simulink model "TunedFuzzy"  (R2024a)
settings: Solver=VariableStepAuto  StartTime=0.0  StopTime=0.24  RelTol=1e-3
InitFcn:
  | fsw = 1e6;
  | Tsw = 1/fsw;
  | 
  | fs = 10e3;%fsw / 4;
  | Ts = 1/fs;
StopFcn:
  | MAE = mean(abs(out.E));
  | Eta = sum((out.P_Pmax{1}.Values.Data))/sum(out.P_Pmax{2}.Values.Data);
undefined symbols (not defined in the file or in its folder): Ion, Lithium, result_Extrapolated_copy
libraries: spsSeriesRLCBranchLib x5, spsCurrentMeasurementLib x4, spsMosfetLib x4, spsVoltageMeasurementLib x3, spsDiodeLib x2, spsBatteryLib x1, spsControlledCurrentSourceLib x1, fuzblock x1, spsPWMGeneratorDCDCLib x1, SignalEditorBlockLib x1, sps_lib x1
settings Model: Creator=kimiaahmadi  LastModifiedBy=kimiaahmadi

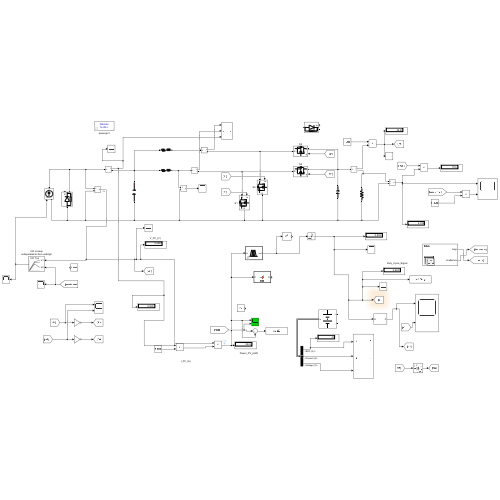
[thumbnail: Simulink's stored preview of the top-level diagram]
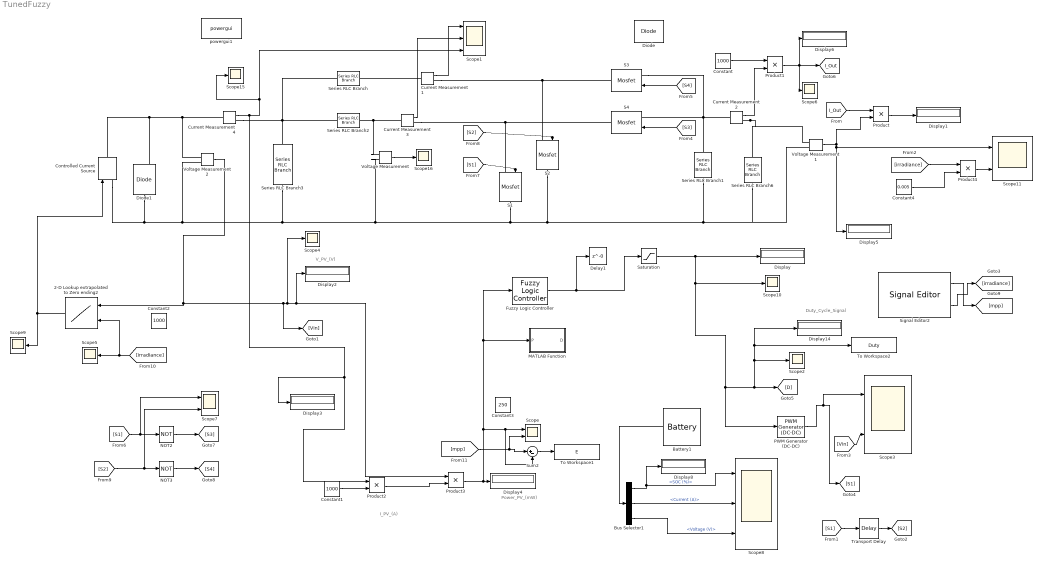
== system TunedFuzzy ==
  note: V_PV_(V)
  note: Duty_Cycle_Signal
  note: I_PV_(A)
  note: Power_PV_(mW)
  2-D Lookup extrapolated to Zero ending2 : Lookup_n-D  BreakpointsForDimension1=[0:7.058900000000000e-04:0.611]  BreakpointsForDimension2=[1:1000]  Table=[result_Extrapolated_copy].'  ExtrapMethod=Clip  UseLastTableValue=on  InternalRulePriority=Speed  RndMeth=Simplest
      settings: InputPortMap=u0,u1
  Battery1 : spsBatteryLib/Battery  BatType=Lithium-Ion  ShowTempParam=off  ThermalPreset=no  ShowAgeParam=off  NomV=3.7  NomQ=0.02  SOC=40  Batt_Tr=0.000001  PresetModel=off  MaxQ=0.03  MinV=3.75  FullV=3.8  Dis_rate=2.3478  R=0.01  Normal_OP=4.8835  expZone="[3.78      0.2653]"  current=[6.5 13 32.5]  Units=Time  Tci=20  NomT=20  T2=-30  MaxQ2=4.8  FullV2=7.1  Normal_OP2=5.655  expZone2="[6.58           1]"  Rca=0.6  ti=2000  Dp=0  Neq0=0  Tsim=1e6  Ta1=25  Qeol=5.4*0.9  Reol=0.013333*1.2  Char_age=[2.3478, 3]  Dis_age=[2.3478, 10]  N1=1500  N2=10500  N3=1000  N4=1400  Ta2=45  N5=950
  Bus Selector1 : BusSelector  OutputSignals=SOC (%),Current (A),Voltage (V)
  Constant : Constant  Value=1000
  Constant1 : Constant  Value=1000
  Constant2 : Constant  Value=1000
  Constant3 : Constant  Value=250
  Constant4 : Constant  Value=0.005
  Controlled Current Source : spsControlledCurrentSourceLib/Controlled Current Source  Initialize=on  Source_Type=AC  Amplitude=0  Phase=0  Frequency=0  Measurements=None
  Current Measurement{1..4} (4 alike) : spsCurrentMeasurementLib/Current Measurement  PhasorSimulation=off  OutputType=Complex  PSBequivalent=0
  Delay1 : Delay  DelayLength=0  InitialCondition=0.9  SampleTime=Ts
  Diode : spsDiodeLib/Diode  Ron=0.001  Lon=0  Vf=0  IC=0  UseSnubber=0  Rs=1e5  Cs=250e-9  Measurements=on
  Diode1 : spsDiodeLib/Diode  Ron=0.001  Lon=0  Vf=0  IC=0  UseSnubber=0  Rs=1e5  Cs=250e-9  Measurements=on
  Display{,1..6,8,14} (9 alike) : Display
  Fuzzy Logic Controller : fuzblock/Fuzzy Logic  Controller  FIS='TunedFuzzyMPPT.fis'  OutputSampleNumber=101  DataType=double  FuzzifiedInputs=off  RuleFiringStrengths=off  RuleOutputs=off  AggregatedOutputs=off  SimulateUsing=Code generation  OutOfRangeInputValueMessage=warning  NoRuleFiredMessage=warning  EmptyOutputFuzzySetMessage=warning
  MATLAB Function : MATLAB Function  TreatAsAtomicUnit=on
  NOT2 : Logic  Operator=NOT  IconShape=distinctive  AllPortsSameDT=off  OutDataTypeStr=boolean
  NOT3 : Logic  Operator=NOT  IconShape=distinctive  AllPortsSameDT=off  OutDataTypeStr=boolean
  PWM Generator (DC-DC) : spsPWMGeneratorDCDCLib/PWM Generator (DC-DC)  Fsw=fsw  Ts=0
  Product{,1..4} (5 alike) : Product
  S{1..4} (4 alike) : spsMosfetLib/Mosfet  Ron=0.1  Lon=0  Rd=0.001  Vfd=0  IC=0  Rs=1e5  Cs=inf  Measurements=off
  Saturation : Saturate  UpperLimit=0.99  LowerLimit=0.01
  Scope{,3,7,11} (4 alike) : Scope  NumInputPorts=2
  Scope1 : Scope  NumInputPorts=3
  Scope{2,4..6,9..10,15..16} (8 alike) : Scope
  Scope8 : Scope  NumInputPorts=3
  Series RLC Branch : spsSeriesRLCBranchLib/Series RLC Branch  LConnTagsString=__new0  RConnTagsString=__new0  BranchType=RL  Resistance=90e-3  Inductance=2.2e-6  SetiL0=off  InitialCurrent=0  Capacitance=1e-6  Setx0=off  InitialVoltage=0  Measurements=None
  Series RLC Branch1 : spsSeriesRLCBranchLib/Series RLC Branch  LConnTagsString=__new0  RConnTagsString=__new0  BranchType=C  Resistance=0  Inductance=1e-3  SetiL0=off  InitialCurrent=0  Capacitance=10e-6  Setx0=off  InitialVoltage=0  Measurements=None
  Series RLC Branch2 : spsSeriesRLCBranchLib/Series RLC Branch  LConnTagsString=__new0  RConnTagsString=__new0  BranchType=RL  Resistance=90e-3  Inductance=2.2e-6  SetiL0=off  InitialCurrent=0  Capacitance=1e-6  Setx0=off  InitialVoltage=0  Measurements=None
  Series RLC Branch3 : spsSeriesRLCBranchLib/Series RLC Branch  LConnTagsString=__new0  RConnTagsString=__new0  BranchType=C  Resistance=1  Inductance=1e-3  SetiL0=off  InitialCurrent=0  Capacitance=10e-6  Setx0=off  InitialVoltage=0  Measurements=None
  Series RLC Branch6 : spsSeriesRLCBranchLib/Series RLC Branch  LConnTagsString=__new0  RConnTagsString=__new0  BranchType=R  Resistance=110  Inductance=1e-3  SetiL0=off  InitialCurrent=0  Capacitance=4700e-6  Setx0=off  InitialVoltage=0  Measurements=None
  Signal Editor2 : SignalEditorBlockLib/Signal Editor  FileName=mpp.mat  ActiveScenario=IEEE  ActiveSignal=mpp  IsBus=off  OutputBusObjectStr=Bus: BusObject  SampleTime=0  ZeroCross=off  OutputAfterFinalValue=Holding final value  Unit=inherit  PreserveSignalName=on  ApplySigPropsToAllScenarios=on  ApplySigPropsToAllSignals=on
  Sum2 : Sum  Inputs=|+-
  To Workspace1 : ToWorkspace  VariableName=E  SampleTime=-1
  To Workspace2 : ToWorkspace  VariableName=Duty  SampleTime=-1
  Transport Delay : TransportDelay  DelayTime=0.5e-6  BufferSize=100
  Voltage Measurement : spsVoltageMeasurementLib/Voltage Measurement  PhasorSimulation=off  OutputType=Complex  PSBequivalent=0
  Voltage Measurement1 : spsVoltageMeasurementLib/Voltage Measurement  PhasorSimulation=off  OutputType=Complex  PSBequivalent=0
  Voltage Measurement2 : spsVoltageMeasurementLib/Voltage Measurement  PhasorSimulation=off  OutputType=Complex  PSBequivalent=0
  powergui1 : sps_lib/powergui  Priority=1  SimulationMode=Discrete  SampleTime=1e-8  frequency=60  Iterations=50  frequencyindice=0  Pbase=100e6  ErrMax=1e-4  UnitsV=kV  UnitsW=MW  buscounter=0  FunctionMessages=off  echomessages=off  EnableUseOfTLC=off  CurrentSourceSwitches=off  DisableSnubberDevices=off  DisableRonSwitches=off  DisableVfSwitches=off  DisplayEquations=off  AutomaticDiscreteSolvers=off  SolverType=Tustin/Backward Euler (TBE)  Interpol=off  ExternalGateDelay=off  methode=off  Ts=100  x0status=blocks  SPID=on  SwTol=0  HookPort=off  NonlinearTolerance=1e-4  nMaxIteration=100  ContinueOnMaxIteration=off  RestoreLinks=warning  ResistiveCurrentMeasurement=off  Frange=[0:2:500]  Ylog=off  Xlog=on  ShowGrid=off  save=off  variable=ZData  structure=0  ZoomFFT=off  StartTime=0.0  cycles=1  DisplayStyle=1  fundamental=60  FreqAxis=off  MaxFrequency=1000  frequencyindicesteady=1  RmsSteady=1  display=off
  tag scope: I_Out=global
  wires:
  Voltage Measurement/1 -> Scope16/1
  Product1/1 -> Scope6/1, Display6/1, [I_Out]
  Current Measurement1/1 -> Scope1/1
  NOT2/1 -> [S3]
  Transport Delay/1 -> [S2]
  [S1] -> Scope7/1, NOT2/1
  [S2] -> S2/1
  PWM Generator (DC-DC)/1 -> [S1], Scope3/1
  Product/1 -> Display1/1
  [S4] -> S3/1
  Bus Selector1/1 -> Scope8/1, Display8/1  "<SOC (%)>"
  Current Measurement3/1 -> Scope1/2
  [S1] -> Transport Delay/1
  [S3] -> S4/1
  [I_Out] -> Product/1
  Bus Selector1/2 -> Scope8/2  "<Current (A)>"
  Current Measurement2/1 -> Product1/2
  NOT3/1 -> [S4]
  [S2] -> Scope7/2, NOT3/1
  Voltage Measurement1/1 -> Display5/1, Scope11/1, Product/2
  Bus Selector1/3 -> Scope8/3  "<Voltage (V)>"
  Battery1/1 -> Bus Selector1/1
  Constant/1 -> Product1/1
  [S1] -> S1/1
  Constant1/1 -> Product2/2
  Product2/1 -> Product3/2
  2-D Lookup extrapolated to Zero ending2/1 -> Scope9/1, Controlled Current Source/1
  [irradiance] -> Product4/1
  Constant4/1 -> Product4/2
  Product4/1 -> Scope11/2
  [Vin] -> Scope3/2
  [mpp] -> Scope/2, Sum2/1
  Voltage Measurement2/1 -> 2-D Lookup extrapolated to Zero ending2/1, [Vin], Scope4/1, Display2/1, Product3/1
  [irradiance] -> 2-D Lookup extrapolated to Zero ending2/2, Scope5/1
  Current Measurement4/1 -> Product2/1, Display3/1, Scope15/1, Scope1/3
  Sum2/1 -> To Workspace1/1
  Saturation/1 -> Scope2/1, Display14/1, To Workspace2/1, [D], PWM Generator (DC-DC)/1, Scope10/1, Display/1
  Product3/1 -> MATLAB Function/1(P), Fuzzy Logic Controller/1, Scope/1, Sum2/2, Display4/1
  Fuzzy Logic Controller/1 -> Saturation/1, Delay1/1
  Signal Editor2/1 -> [mpp]
  Signal Editor2/2 -> [irradiance]
  connections:
  Controlled Current Source/LConn1 -- Diode1/LConn1 -- Voltage Measurement2/LConn2 -- Series RLC Branch3/RConn1 -- Voltage Measurement/LConn2 -- S1/RConn1 -- Voltage Measurement1/LConn2 -- Series RLC Branch6/RConn1 -- Series RLC Branch1/RConn1 -- S2/RConn1
  Current Measurement2/LConn1 -- S3/LConn1 -- S4/LConn1 -- Series RLC Branch1/LConn1
  Current Measurement4/RConn1 -- Series RLC Branch3/LConn1 -- Series RLC Branch/LConn1 -- Series RLC Branch2/LConn1
  Current Measurement3/LConn1 -- Voltage Measurement/LConn1 -- Series RLC Branch2/RConn1
  S1/LConn1 -- S4/RConn1 -- Current Measurement3/RConn1
  Controlled Current Source/RConn1 -- Diode1/RConn1 -- Voltage Measurement2/LConn1 -- Current Measurement4/LConn1
  S2/LConn1 -- S3/RConn1 -- Current Measurement1/RConn1
  Current Measurement2/RConn1 -- Voltage Measurement1/LConn1 -- Series RLC Branch6/LConn1
  Current Measurement1/LConn1 -- Series RLC Branch/RConn1

== matlab function TunedFuzzy/MATLAB Function ==
  data: P input; D output
function D = fcn(P)

% fis = readfis('TunedFuzzyMPPT.fis');
fis = getFISCodeGenerationData('TunedFuzzyMPPT.fis');
D = evalfis(fis,P);
